simulink model "lab_5_simulink"  (R2024a)
settings: Solver=ode4  StartTime=0.0  StopTime=100.0  FixedStep=1/64  RelTol=1e-3
settings Model: Creator=lw53894  LastModifiedBy=lw53894

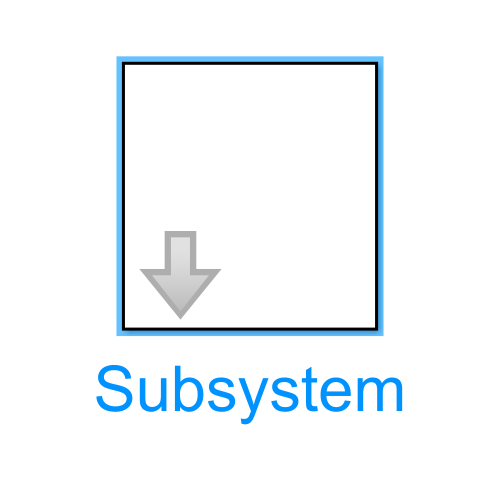
[thumbnail: Simulink's stored preview of the top-level diagram]
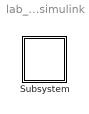
== system lab_5_simulink ==
  Subsystem : Subsystem  mask{g=9.81, l=1.5, m=3, k=5, r0=2, r_prim_0=1, o0=45, o_prim_0=12}

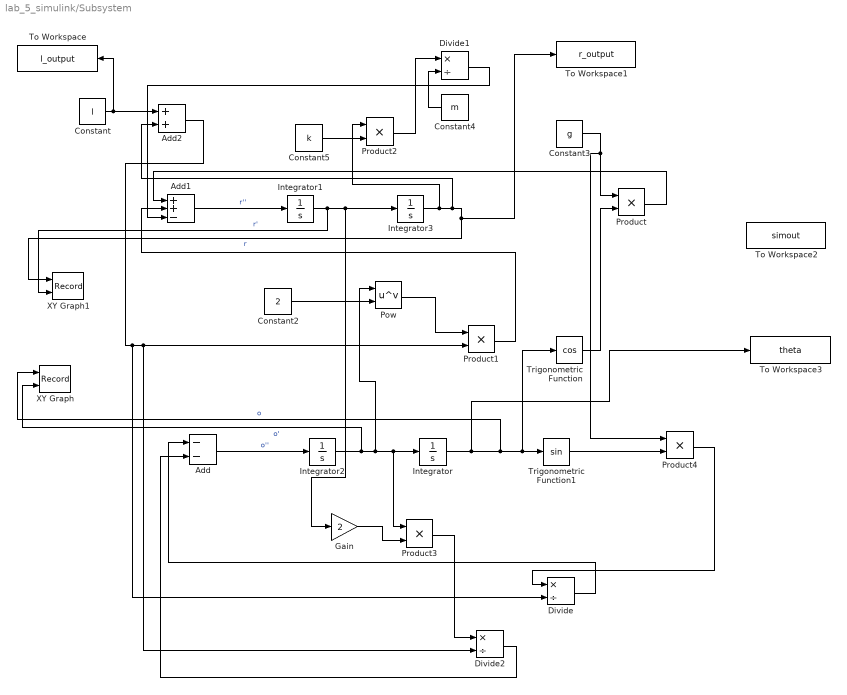
== system lab_5_simulink/Subsystem ==
  Add : Sum  Inputs=--
  Add1 : Sum  Inputs=++-
  Add2 : Sum
  Constant : Constant  Value=l
  Constant2 : Constant  Value=2
  Constant3 : Constant  Value=g
  Constant4 : Constant  Value=m
  Constant5 : Constant  Value=k
  Divide : Product  Inputs=*/
  Divide1 : Product  Inputs=*/
  Divide2 : Product  Inputs=*/
  Gain : Gain  Gain=2
  Integrator : Integrator  InitialCondition=(o0*pi)/180
  Integrator1 : Integrator  InitialCondition=r_prim_0
  Integrator2 : Integrator  InitialCondition=(o_prim_0*pi)/180
  Integrator3 : Integrator  InitialCondition=r0
  Pow : Math  Operator=pow  SignedPower=on  RndMeth=Zero
  Product{,1..4} (5 alike) : Product
  To Workspace : ToWorkspace  VariableName=l_output  SaveFormat=Timeseries  SampleTime=-1
  To Workspace1 : ToWorkspace  VariableName=r_output  SaveFormat=Timeseries  SampleTime=-1
  To Workspace2 : ToWorkspace  VariableName=simout  SaveFormat=Timeseries  SampleTime=-1
  To Workspace3 : ToWorkspace  VariableName=theta  SaveFormat=Timeseries  SampleTime=-1
  Trigonometric Function : Trigonometry  Operator=cos
  Trigonometric Function1 : Trigonometry
  XY Graph : Record  FileSettingsInternal="{\"entries\":[{\"content\":{\"excelSettings\":{\"content\":{},\"type\":\"Streamout.ExcelSettings\"}},\"type\":\"Streamout.FileSettingStorage\",\"uuid\":\"\"}],\"packageUris\":[\"http:\\/\\/schema.mathworks.com\\/mf0\\/streamout_blocks\\/R2020a\"],\"version\":\"1.0\"}"  Layout=[1 1]  SignalsInternal="{\"entries\":[{\"content\":{\"signals\":[{\"content\":{\"blockPath\":[],\"dimensions\":[1],\"domain\":\"\",\"lineColor\":\"#a2142f\",\"plots\":[ 1 ],\"port\":1,\"sid\":[\"\"],\"signalID\":1,\"signalName\":\"o\"},\"type\":\"RecordBlkView.Signal\",\"uuid\":\"\"},{\"content\":{\"blockPath\":[],\"dimensions\":[1],\"domain\":\"\",\"lineColor\":\"#139fff\",\"plots\":[ 1 ],\"port\":2,\"sid\":[\"\"],\"signalID\":2,\"signalName\":\"o'\"},\"type\":\"RecordBlkView.Signal\",\"uuid\":\"\"}]},\"type\":\"RecordBlkView.InputSignals\",\"uuid\":\"\"}],\"packageUris\":[\"http:\\/\\/schema.mathworks.com\\/mf0\\/streamout_blocks\\/R2020a\"],\"version\":\"1.0\"}"  VisualizationBindings="{\"xyplotplugin\":{\"info\":[{\"series\":[{\"bindingParametersList\":[{\"parameter\":\"X-Axis\",\"signalID\":1,\"signalName\":\"o\"},{\"parameter\":\"Y-Axis\",\"signalID\":2,\"signalName\":\"o'\"}],\"seriesID\":0}],\"subplotID\":1}]}}"  CompatibilityTag=XY
  XY Graph1 : Record  FileSettingsInternal="{\"entries\":[{\"content\":{\"excelSettings\":{\"content\":{},\"type\":\"Streamout.ExcelSettings\"}},\"type\":\"Streamout.FileSettingStorage\",\"uuid\":\"\"}],\"packageUris\":[\"http:\\/\\/schema.mathworks.com\\/mf0\\/streamout_blocks\\/R2020a\"],\"version\":\"1.0\"}"  Layout=[1 1]  SignalsInternal="{\"entries\":[{\"content\":{\"signals\":[{\"content\":{\"blockPath\":[],\"dimensions\":[1],\"domain\":\"\",\"lineColor\":\"#a2142f\",\"plots\":[ 1 ],\"port\":1,\"sid\":[\"\"],\"signalID\":1,\"signalName\":\"r\"},\"type\":\"RecordBlkView.Signal\",\"uuid\":\"\"},{\"content\":{\"blockPath\":[],\"dimensions\":[1],\"domain\":\"\",\"lineColor\":\"#139fff\",\"plots\":[ 1 ],\"port\":2,\"sid\":[\"\"],\"signalID\":2,\"signalName\":\"r'\"},\"type\":\"RecordBlkView.Signal\",\"uuid\":\"\"}]},\"type\":\"RecordBlkView.InputSignals\",\"uuid\":\"\"}],\"packageUris\":[\"http:\\/\\/schema.mathworks.com\\/mf0\\/streamout_blocks\\/R2020a\"],\"version\":\"1.0\"}"  VisualizationBindings="{\"xyplotplugin\":{\"info\":[{\"series\":[{\"bindingParametersList\":[{\"parameter\":\"X-Axis\",\"signalID\":1,\"signalName\":\"r\"},{\"parameter\":\"Y-Axis\",\"signalID\":2,\"signalName\":\"r'\"}],\"seriesID\":0}],\"subplotID\":1}]}}"  CompatibilityTag=XY
  wires:
  Pow/1 -> Product1/1
  Integrator2/1 -> XY Graph/2, Pow/1, Product3/1, Integrator/1  "o'"
  Product1/1 -> Add1/2
  Constant4/1 -> Divide1/2
  Add1/1 -> Integrator1/1  "r''"
  Integrator3/1 -> Product2/1, Add2/2, To Workspace1/1, XY Graph1/1  "r"
  Integrator1/1 -> XY Graph1/2, Integrator3/1, Gain/1  "r'"
  Add/1 -> Integrator2/1  "o''"
  Constant/1 -> To Workspace/1, Add2/1
  Divide1/1 -> Add1/3
  Product/1 -> Add1/1
  Add2/1 -> Divide/2, Divide2/2, Product1/2
  Constant2/1 -> Pow/2
  Gain/1 -> Product3/2
  Constant3/1 -> Product4/1, Product/1
  Trigonometric Function/1 -> Product/2
  Integrator/1 -> To Workspace3/1, XY Graph/1, Trigonometric Function/1, Trigonometric Function1/1  "o"
  Constant5/1 -> Product2/2
  Product2/1 -> Divide1/1
  Divide/1 -> Add/1
  Product3/1 -> Divide2/1
  Divide2/1 -> Add/2
  Trigonometric Function1/1 -> Product4/2
  Product4/1 -> Divide/1
